simulink library "tp333079"  (Simulink 5.0)
values from neighbouring files (symbols this model uses):
  b = 1    [main_flock3.m]    (also in main_flock4.m; params_flocking_ros.m)
undefined symbols (not defined in the file or in its folder): AC, AlphaBnd, BetaBnd, CDda, CDde, CDdf, CDdr, CDM, CDmin, CGempty, CGgross, CL0, CLa, CLalphadot, Clbeta, Clda, CLde, CLdf, Cldr, CLM, CLmind, Clp, CLq, Clr, Cm0, Cma, Cmalphadot, Cmde, Cmdf, CmM, Cmq, Cnbeta, Cnda, Cndr, Cnp, Cnr, CP, CT, CYbeta, CYda, CYdr, CYp, CYr, Displacement, dmy, Engine, EulerIni, FuelFlow, FuelIni, J, Jempty, Jeng, Jgross, Jprop, MAC, MAP, MAPLim, MassIni, MaxPower, mempty ... (+26)
libraries: aerosimlib x325, simulink3 x42
(part 7 of 11)

== system tp333079/Equations of Motion/Geodetic-Frame EOM/Position ==
  note: Sources
  note: Position derivatives
  note: Navigation equation
  Vel NED : Inport  Port=1  PortDimensions=[3 1]  SampleTime=-1  DataType=auto
      settings: SignalType=auto
  Rmeridian : Inport  Port=2  PortDimensions=1  SampleTime=-1  DataType=auto
      settings: SignalType=auto
  Rnormal : Inport  Port=3  PortDimensions=1  SampleTime=-1  DataType=auto
      settings: SignalType=auto
  AConGnd : Inport  Port=4  PortDimensions=1  SampleTime=-1  DataType=auto
      settings: SignalType=auto
  RST : Inport  Port=5  PortDimensions=1  SampleTime=-1  DataType=auto
      settings: SignalType=auto
  Altitude Switch : Switch  Threshold=1
  ChSign : Gain  Gain=-1  Multiplication=Element-wise(K.*u)  SaturateOnIntegerOverflow=on
  Demux1 : Demux  Outputs=3  BusSelectionMode=off
  Demux3 : Demux  Outputs=3  BusSelectionMode=off
  Latitude Bound : Subsystem  SimViewingDevice=off
      settings: Permissions=ReadWrite  RTWFcnNameOpts=Auto  RTWFileNameOpts=Auto
      mask Type: Latitude bound
      mask Description: Bounds the latitude to [-pi/2, pi/2]. When the lower bound is exceeded the latitude is increasing again; when the upper bound is exceeded the latitude is decreasing.
  Longitude Bound : Subsystem  SimViewingDevice=off
      settings: Permissions=ReadWrite  RTWFcnNameOpts=Auto  RTWFileNameOpts=Auto
      mask Type: Longitude bound
      mask Description: Bounds the longitude to [-pi, pi]. When -pi bound is exceeded the longitude wraps back to pi; when the pi bound is exceeded the longitude wraps back to -pi.
  Mux : Mux  Inputs=3
  Mux1 : Mux  Inputs=3
  Position Integrator : Integrator  ExternalReset=rising  InitialConditionSource=internal  InitialCondition=PositionIni  LimitOutput=off  UpperSaturationLimit=inf  LowerSaturationLimit=-inf  ShowSaturationPort=off  ShowStatePort=off  AbsoluteTolerance=auto
  Sum : Sum  Inputs=|++  SaturateOnIntegerOverflow=on
  Sum1 : Sum  Inputs=|++  SaturateOnIntegerOverflow=on
  Ve/(Rn+h)cos(phi) : Product  Inputs=*//  Multiplication=Element-wise(.*)  SaturateOnIntegerOverflow=on
  Vn/(Rm+h) : Product  Inputs=*/  Multiplication=Element-wise(.*)  SaturateOnIntegerOverflow=on
  Zero : Constant  Value=0
  cos(phi) : Trigonometry  Operator=cos  OutputSignalType=auto
  Position : Outport  Port=1
  dPosdt : Outport  Port=2
  wires:
  Demux1/1 -> Vn/(Rm+h)/1
  Demux1/3 -> ChSign/1
  Demux1/2 -> Ve/(Rn+h)cos(phi)/1
  Vel NED/1 -> Demux1/1
  Rmeridian/1 -> Sum/1
  Rnormal/1 -> Sum1/1
  Sum/1 -> Vn/(Rm+h)/2
  Vn/(Rm+h)/1 -> Mux/1
  Sum1/1 -> Ve/(Rn+h)cos(phi)/2
  Ve/(Rn+h)cos(phi)/1 -> Mux/2
  AConGnd/1 -> Altitude Switch/2
  Zero/1 -> Altitude Switch/1
  ChSign/1 -> Altitude Switch/3
  Altitude Switch/1 -> Mux/3
  Mux/1 -> Position Integrator/1, dPosdt/1
  RST/1 -> Position Integrator/2
  Position Integrator/1 -> Demux3/1
  cos(phi)/1 -> Ve/(Rn+h)cos(phi)/3
  Demux3/3 -> Sum/2, Sum1/2, Mux1/3
  Demux3/2 -> Longitude Bound/1(In)
  Demux3/1 -> Latitude Bound/1(In)
  Longitude Bound/1(Out) -> Mux1/2
  Mux1/1 -> Position/1
  Latitude Bound/1(Out) -> cos(phi)/1, Mux1/1

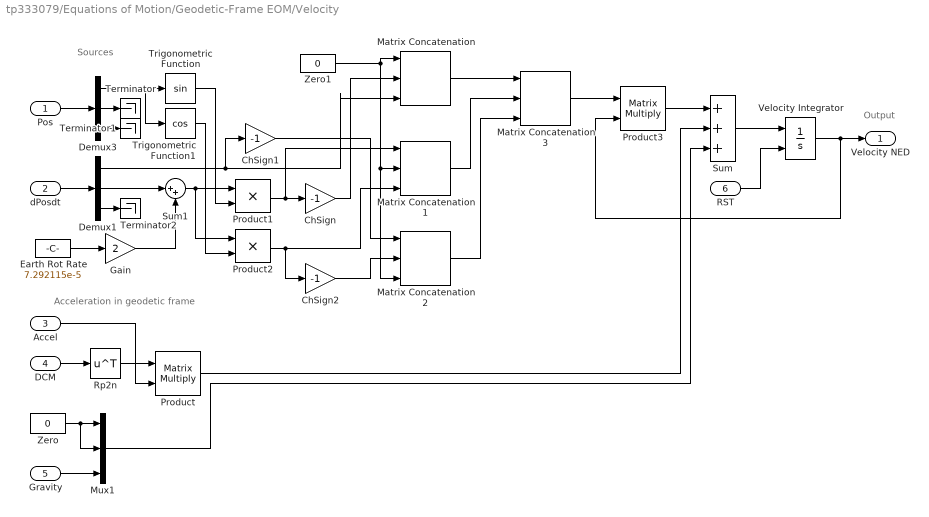
== system tp333079/Equations of Motion/Geodetic-Frame EOM/Velocity ==
  note: Sources
  note: Output
  note: Acceleration in geodetic frame
  Pos : Inport  Port=1  PortDimensions=[3 1]  SampleTime=-1  DataType=auto
      settings: SignalType=auto
  dPosdt : Inport  Port=2  PortDimensions=[3 1]  SampleTime=-1  DataType=auto
      settings: SignalType=auto
  Accel : Inport  Port=3  PortDimensions=[3 1]  SampleTime=-1  DataType=auto
      settings: SignalType=auto
  DCM : Inport  Port=4  PortDimensions=[3 3]  SampleTime=-1  DataType=auto
      settings: SignalType=auto
  Gravity : Inport  Port=5  PortDimensions=1  SampleTime=-1  DataType=auto
      settings: SignalType=auto
  RST : Inport  Port=6  PortDimensions=1  SampleTime=-1  DataType=auto
      settings: SignalType=auto
  ChSign : Gain  Gain=-1  Multiplication=Element-wise(K.*u)  SaturateOnIntegerOverflow=on
  ChSign1 : Gain  Gain=-1  Multiplication=Element-wise(K.*u)  SaturateOnIntegerOverflow=on
  ChSign2 : Gain  Gain=-1  Multiplication=Element-wise(K.*u)  SaturateOnIntegerOverflow=on
  Demux1 : Demux  Outputs=3  BusSelectionMode=off
  Demux3 : Demux  Outputs=3  BusSelectionMode=off
  Earth Rot Rate : Constant  Value=7.292115e-5
  Gain : Gain  Gain=2  Multiplication=Element-wise(K.*u)  SaturateOnIntegerOverflow=on
  Matrix Concatenation : simulink3/Signals & Systems/Matrix Concatenation  numInports=3  catMethod=Horizontal
  Matrix Concatenation1 : simulink3/Signals & Systems/Matrix Concatenation  numInports=3  catMethod=Horizontal
  Matrix Concatenation2 : simulink3/Signals & Systems/Matrix Concatenation  numInports=3  catMethod=Horizontal
  Matrix Concatenation3 : simulink3/Signals & Systems/Matrix Concatenation  numInports=3  catMethod=Vertical
  Mux1 : Mux  Inputs=3
  Product : Product  Inputs=2  Multiplication=Matrix(*)  SaturateOnIntegerOverflow=on
  Product1 : Product  Inputs=2  Multiplication=Element-wise(.*)  SaturateOnIntegerOverflow=on
  Product2 : Product  Inputs=2  Multiplication=Element-wise(.*)  SaturateOnIntegerOverflow=on
  Product3 : Product  Inputs=2  Multiplication=Matrix(*)  SaturateOnIntegerOverflow=on
  Rp2n : Math  Operator=transpose  OutputSignalType=auto
  Sum : Sum  Inputs=+++  SaturateOnIntegerOverflow=on
  Sum1 : Sum  Inputs=|++  SaturateOnIntegerOverflow=on
  Terminator : Terminator
  Terminator1 : Terminator
  Terminator2 : Terminator
  Trigonometric Function : Trigonometry  Operator=sin  OutputSignalType=auto
  Trigonometric Function1 : Trigonometry  Operator=cos  OutputSignalType=auto
  Velocity Integrator : Integrator  ExternalReset=rising  InitialConditionSource=internal  InitialCondition=VelocitiesIni  LimitOutput=off  UpperSaturationLimit=inf  LowerSaturationLimit=-inf  ShowSaturationPort=off  ShowStatePort=off  AbsoluteTolerance=auto
  Zero : Constant  Value=0
  Zero1 : Constant  Value=0
  Velocity NED : Outport  Port=1
  wires:
  Zero/1 -> Mux1/2, Mux1/1
  Gravity/1 -> Mux1/3
  Sum/1 -> Velocity Integrator/1
  RST/1 -> Velocity Integrator/2
  Velocity Integrator/1 -> Velocity NED/1, Product3/2
  DCM/1 -> Rp2n/1
  Rp2n/1 -> Product/1
  Accel/1 -> Product/2
  Pos/1 -> Demux3/1
  dPosdt/1 -> Demux1/1
  Earth Rot Rate/1 -> Gain/1
  Demux1/2 -> Sum1/1
  Gain/1 -> Sum1/2
  Demux3/1 -> Trigonometric Function/1, Trigonometric Function1/1
  Sum1/1 -> Product1/1, Product2/1
  Trigonometric Function/1 -> Product1/2
  Trigonometric Function1/1 -> Product2/2
  Zero1/1 -> Matrix Concatenation/1, Matrix Concatenation1/2, Matrix Concatenation2/3
  Product1/1 -> ChSign/1, Matrix Concatenation1/1
  ChSign/1 -> Matrix Concatenation/2
  Demux1/1 -> Matrix Concatenation/3, ChSign1/1
  Product2/1 -> Matrix Concatenation1/3, ChSign2/1
  ChSign1/1 -> Matrix Concatenation2/1
  ChSign2/1 -> Matrix Concatenation2/2
  Demux3/2 -> Terminator/1
  Demux3/3 -> Terminator1/1
  Demux1/3 -> Terminator2/1
  Matrix Concatenation/1 -> Matrix Concatenation3/1
  Matrix Concatenation1/1 -> Matrix Concatenation3/2
  Matrix Concatenation2/1 -> Matrix Concatenation3/3
  Matrix Concatenation3/1 -> Product3/1
  Product3/1 -> Sum/1
  Product/1 -> Sum/2
  Mux1/1 -> Sum/3

== system tp333079/Equations of Motion/Total Moment/Aero Moment ==
  Vec1 : Inport  Port=1  PortDimensions=-1  SampleTime=-1  DataType=auto
      settings: SignalType=auto
  Vec2 : Inport  Port=2  PortDimensions=-1  SampleTime=-1  DataType=auto
      settings: SignalType=auto
  Product : Product  Inputs=2  Multiplication=Element-wise(.*)  SaturateOnIntegerOverflow=on
  Product1 : Product  Inputs=2  Multiplication=Element-wise(.*)  SaturateOnIntegerOverflow=on
  Selector : Selector  InputType=Vector  ElementSrc=Internal  Elements=[2 3 1]  RowSrc=Internal  Rows=1  ColumnSrc=Internal  Columns=1  InputPortWidth=3
  Selector1 : Selector  InputType=Vector  ElementSrc=Internal  Elements=[3 1 2]  RowSrc=Internal  Rows=1  ColumnSrc=Internal  Columns=1  InputPortWidth=3
  Selector2 : Selector  InputType=Vector  ElementSrc=Internal  Elements=[3 1 2]  RowSrc=Internal  Rows=1  ColumnSrc=Internal  Columns=1  InputPortWidth=3
  Selector3 : Selector  InputType=Vector  ElementSrc=Internal  Elements=[2 3 1]  RowSrc=Internal  Rows=1  ColumnSrc=Internal  Columns=1  InputPortWidth=3
  Sum : Sum  Inputs=+-  SaturateOnIntegerOverflow=on
  ProdVec : Outport  Port=1
  wires:
  Sum/1 -> ProdVec/1
  Product1/1 -> Sum/2
  Product/1 -> Sum/1
  Selector3/1 -> Product1/2
  Selector2/1 -> Product1/1
  Selector1/1 -> Product/2
  Selector/1 -> Product/1
  Vec2/1 -> Selector3/1, Selector1/1
  Vec1/1 -> Selector2/1, Selector/1

== system tp333079/Equations of Motion/Total Moment/Propulsion Moment ==
  Vec1 : Inport  Port=1  PortDimensions=-1  SampleTime=-1  DataType=auto
      settings: SignalType=auto
  Vec2 : Inport  Port=2  PortDimensions=-1  SampleTime=-1  DataType=auto
      settings: SignalType=auto
  Product : Product  Inputs=2  Multiplication=Element-wise(.*)  SaturateOnIntegerOverflow=on
  Product1 : Product  Inputs=2  Multiplication=Element-wise(.*)  SaturateOnIntegerOverflow=on
  Selector : Selector  InputType=Vector  ElementSrc=Internal  Elements=[2 3 1]  RowSrc=Internal  Rows=1  ColumnSrc=Internal  Columns=1  InputPortWidth=3
  Selector1 : Selector  InputType=Vector  ElementSrc=Internal  Elements=[3 1 2]  RowSrc=Internal  Rows=1  ColumnSrc=Internal  Columns=1  InputPortWidth=3
  Selector2 : Selector  InputType=Vector  ElementSrc=Internal  Elements=[3 1 2]  RowSrc=Internal  Rows=1  ColumnSrc=Internal  Columns=1  InputPortWidth=3
  Selector3 : Selector  InputType=Vector  ElementSrc=Internal  Elements=[2 3 1]  RowSrc=Internal  Rows=1  ColumnSrc=Internal  Columns=1  InputPortWidth=3
  Sum : Sum  Inputs=+-  SaturateOnIntegerOverflow=on
  ProdVec : Outport  Port=1
  wires:
  Vec1/1 -> Selector/1, Selector2/1
  Vec2/1 -> Selector1/1, Selector3/1
  Selector/1 -> Product/1
  Selector1/1 -> Product/2
  Selector2/1 -> Product1/1
  Selector3/1 -> Product1/2
  Product/1 -> Sum/1
  Product1/1 -> Sum/2
  Sum/1 -> ProdVec/1

== system tp333079/FlightGear-Compatible/Aerodynamics/Coefficient ==
  RowParam : Inport  Port=1  PortDimensions=-1  SampleTime=-1  DataType=auto
      settings: SignalType=auto
  ColParam : Inport  Port=2  PortDimensions=-1  SampleTime=-1  DataType=auto
      settings: SignalType=auto
  Value : aerosimlib/FlightGear-Compatible/Aerodynamics/Value  Value=0
  term2 : Terminator
  Coeff : Outport  Port=1
  wires:
  RowParam/1 -> Value/1
  Value/1 -> Coeff/1
  ColParam/1 -> term2/1

== system tp333079/FlightGear-Compatible/Aerodynamics/Table ==
  RowParam : Inport  Port=1  PortDimensions=-1  SampleTime=-1  DataType=auto
      settings: SignalType=auto
  ColParam : Inport  Port=2  PortDimensions=-1  SampleTime=-1  DataType=auto
      settings: SignalType=auto
  Look-Up Table (2-D) : Lookup2D  RowIndex=Table.RowArg  ColumnIndex=Table.ColArg  OutputValues=Table.Data
  Coeff : Outport  Port=1
  wires:
  Look-Up Table (2-D)/1 -> Coeff/1
  ColParam/1 -> Look-Up Table (2-D)/2
  RowParam/1 -> Look-Up Table (2-D)/1

== system tp333079/FlightGear-Compatible/Aerodynamics/Value ==
  RowParam : Inport  Port=1  PortDimensions=-1  SampleTime=-1  DataType=auto
      settings: SignalType=auto
  Gain : Gain  Gain=Value.Data  Multiplication=Element-wise(K.*u)  SaturateOnIntegerOverflow=on
  Coeff : Outport  Port=1
  wires:
  RowParam/1 -> Gain/1
  Gain/1 -> Coeff/1

== system tp333079/FlightGear-Compatible/Aerodynamics/Vector ==
  RowParam : Inport  Port=1  PortDimensions=-1  SampleTime=-1  DataType=auto
      settings: SignalType=auto
  Look-Up Table : Lookup  InputValues=Vector.RowArg  OutputValues=Vector.Data
  Coeff : Outport  Port=1
  wires:
  RowParam/1 -> Look-Up Table/1
  Look-Up Table/1 -> Coeff/1

== system tp333079/FlightGear-Compatible/Complete Aircraft/CESSNA-172 ==
  Control : Inport  Port=1  PortDimensions=[7 1]  SampleTime=-1  DataType=auto
      settings: SignalType=auto
  Wind : Inport  Port=2  PortDimensions=[3 1]  SampleTime=-1  DataType=auto
      settings: SignalType=auto
  RST : Inport  Port=3  PortDimensions=1  SampleTime=-1  DataType=auto
      settings: SignalType=auto
  Aerodynamics : Subsystem  SimViewingDevice=off
      settings: Permissions=ReadWrite  RTWFcnNameOpts=Auto  RTWFileNameOpts=Auto
  Aircraft Inertia : Subsystem  SimViewingDevice=off
      settings: Permissions=ReadWrite  RTWFcnNameOpts=Auto  RTWFileNameOpts=Auto
  Atmosphere : Subsystem  SimViewingDevice=off
      settings: Permissions=ReadWrite  RTWFcnNameOpts=Auto  RTWFileNameOpts=Auto
  Demux : Demux  Outputs=7  BusSelectionMode=off
  Demux1 : Demux  Outputs=3  BusSelectionMode=off
  Earth : Subsystem  SimViewingDevice=off
      settings: Permissions=ReadWrite  RTWFcnNameOpts=Auto  RTWFileNameOpts=Auto
  Equations of Motion : Subsystem  SimViewingDevice=off
      settings: Permissions=ReadWrite  RTWFcnNameOpts=Auto  RTWFileNameOpts=Auto
  F/m : Product  Inputs=*/  Multiplication=Element-wise(.*)  SaturateOnIntegerOverflow=on
  Mux : Mux  Inputs=4
  Mux1 : Mux  Inputs=3
  Propulsion System : aerosimlib/FlightGear-Compatible/Propulsion/FG Piston Engine +  Fixed-Pitch Prop  Eng=AC.Propulsion.Engine{1}  Thr=AC.Propulsion.Thruster{1}  pSL=101325  TSL=288.15  OmegaIni=OmegaIni
  Sum1 : Sum  Inputs=++  SaturateOnIntegerOverflow=on
  Sum2 : Sum  Inputs=++  SaturateOnIntegerOverflow=on
  rad/s 2 RPM : aerosimlib/Unit Conversion/Angular velocity/rad//s 2 RPM
  TAS : Outport  Port=1
  AOA : Outport  Port=2
  Position : Outport  Port=3
  Attitude : Outport  Port=4
  Rates : Outport  Port=5
  Aero : Outport  Port=6
  Prop : Outport  Port=7
  Engine : Outport  Port=8
  RPM : Outport  Port=9
  wires:
  rad/s 2 RPM/1 -> RPM/1
  Propulsion System/3 -> rad/s 2 RPM/1
  Propulsion System/5 -> Engine/1
  Propulsion System/6 -> Prop/1
  Aerodynamics/3(AeroCoeff) -> Aero/1
  Equations of Motion/7(Euler) -> Attitude/1
  Demux1/3 -> AOA/1
  Demux1/1 -> TAS/1
  Equations of Motion/6(DCM) -> Atmosphere/6(DCM)
  Equations of Motion/1(VelB) -> Atmosphere/4(VelB), Aerodynamics/2(VelB)
  Equations of Motion/3(Rates) -> Rates/1, Aerodynamics/4(Rates)
  Earth/2(AGL) -> Aerodynamics/8(AGL), Atmosphere/2(AGL)
  Earth/1(MSL) -> Atmosphere/1(MSL)
  Earth/3(AConGnd) -> Equations of Motion/6(AConGnd)
  Earth/6(Gravity) -> Equations of Motion/5(Gravity)
  Earth/4(Rearth) -> Equations of Motion/4(Rearth)
  Equations of Motion/5(Pos) -> Position/1, Earth/1(Position)
  Aircraft Inertia/3(Inertia) -> Equations of Motion/3(Inertia)
  Aircraft Inertia/2(CG) -> Propulsion System/6, Aerodynamics/9(CGpos)
  Aircraft Inertia/1(Mass) -> F/m/2
  Propulsion System/4 -> Aircraft Inertia/1(FuelFlow)
  RST/1 -> Aircraft Inertia/2(RST), Equations of Motion/7(RST), Propulsion System/7
  Aerodynamics/4(VelW) -> Demux1/1, Atmosphere/5(VelW), Propulsion System/5
  Atmosphere/2(OAT) -> Propulsion System/3
  Atmosphere/1(pstatic) -> Propulsion System/2
  Atmosphere/5(WindVel) -> Aerodynamics/3(WindB)
  Atmosphere/6(WindRates) -> Aerodynamics/5(WindRates)
  Wind/1 -> Atmosphere/3(Winds)
  Atmosphere/4(a) -> Aerodynamics/7(a)
  Atmosphere/3(rho) -> Propulsion System/4, Aerodynamics/6(rho)
  Mux1/1 -> Propulsion System/1
  Mux/1 -> Aerodynamics/1(Control)
  Control/1 -> Demux/1
  Demux/7 -> Mux1/3
  Demux/6 -> Mux1/2
  Demux/5 -> Mux1/1
  Demux/4 -> Mux/4
  Demux/3 -> Mux/3
  Demux/2 -> Mux/2
  Demux/1 -> Mux/1
  F/m/1 -> Equations of Motion/1(Accel)
  Sum2/1 -> F/m/1
  Sum1/1 -> Equations of Motion/2(Moment)
  Aerodynamics/1(Faero) -> Sum2/1
  Propulsion System/1 -> Sum2/2
  Propulsion System/2 -> Sum1/2
  Aerodynamics/2(Maero) -> Sum1/1

== system tp333079/FlightGear-Compatible/Complete Aircraft/CESSNA-182 ==
  Control : Inport  Port=1  PortDimensions=[8 1]  SampleTime=-1  DataType=auto
      settings: SignalType=auto
  Wind : Inport  Port=2  PortDimensions=[3 1]  SampleTime=-1  DataType=auto
      settings: SignalType=auto
  RST : Inport  Port=3  PortDimensions=1  SampleTime=-1  DataType=auto
      settings: SignalType=auto
  Aerodynamics : Subsystem  SimViewingDevice=off
      settings: Permissions=ReadWrite  RTWFcnNameOpts=Auto  RTWFileNameOpts=Auto
  Aircraft Inertia : Subsystem  SimViewingDevice=off
      settings: Permissions=ReadWrite  RTWFcnNameOpts=Auto  RTWFileNameOpts=Auto
  Atmosphere : aerosimlib/FlightGear-Compatible/Complete Aircraft/CESSNA-172/Atmosphere  SimViewingDevice=off
      settings: Permissions=ReadWrite  RTWFcnNameOpts=Auto  RTWFileNameOpts=Auto
  Demux : Demux  Outputs=8  BusSelectionMode=off
  Demux1 : Demux  Outputs=3  BusSelectionMode=off
  Earth : Subsystem  SimViewingDevice=off
      settings: Permissions=ReadWrite  RTWFcnNameOpts=Auto  RTWFileNameOpts=Auto
  Equations of Motion : Subsystem  SimViewingDevice=off
      settings: Permissions=ReadWrite  RTWFcnNameOpts=Auto  RTWFileNameOpts=Auto
  F/m : Product  Inputs=*/  Multiplication=Element-wise(.*)  SaturateOnIntegerOverflow=on
  FG Piston Engine +  Variable-Pitch Prop : aerosimlib/FlightGear-Compatible/Propulsion/FG Piston Engine +  Variable-Pitch Prop  Eng=AC.Propulsion.Engine{1}  Thr=AC.Propulsion.Thruster{1}  pSL=101325  TSL=288.15  OmegaIni=OmegaIni
  Mux : Mux  Inputs=4
  Mux1 : Mux  Inputs=4
  Sum1 : Sum  Inputs=++  SaturateOnIntegerOverflow=on
  Sum2 : Sum  Inputs=++  SaturateOnIntegerOverflow=on
  rad/s 2 RPM : aerosimlib/Unit Conversion/Angular velocity/rad//s 2 RPM
  TAS : Outport  Port=1
  AOA : Outport  Port=2
  Position : Outport  Port=3
  Attitude : Outport  Port=4
  Rates : Outport  Port=5
  Aero : Outport  Port=6
  Prop : Outport  Port=7
  Engine : Outport  Port=8
  RPM : Outport  Port=9
  wires:
  Demux/8 -> Mux1/4
  rad/s 2 RPM/1 -> RPM/1
  FG Piston Engine +  Variable-Pitch Prop/3 -> rad/s 2 RPM/1
  FG Piston Engine +  Variable-Pitch Prop/5 -> Engine/1
  FG Piston Engine +  Variable-Pitch Prop/6 -> Prop/1
  Aerodynamics/3(AeroCoeff) -> Aero/1
  Equations of Motion/7(Euler) -> Attitude/1
  Demux1/3 -> AOA/1
  Demux1/1 -> TAS/1
  Equations of Motion/6(DCM) -> Atmosphere/6
  Equations of Motion/1(VelB) -> Aerodynamics/2(VelB), Atmosphere/4
  Equations of Motion/3(Rates) -> Rates/1, Aerodynamics/4(Rates)
  Earth/2(AGL) -> Aerodynamics/8(AGL), Atmosphere/2
  Earth/1(MSL) -> Atmosphere/1
  Earth/3(AConGnd) -> Equations of Motion/6(AConGnd)
  Earth/6(Gravity) -> Equations of Motion/5(Gravity)
  Earth/4(Rearth) -> Equations of Motion/4(Rearth)
  Equations of Motion/5(Pos) -> Position/1, Earth/1(Position)
  Aircraft Inertia/3(Inertia) -> Equations of Motion/3(Inertia)
  F/m/1 -> Equations of Motion/1(Accel)
  Aircraft Inertia/2(CG) -> FG Piston Engine +  Variable-Pitch Prop/6, Aerodynamics/9(CGpos)
  Aircraft Inertia/1(Mass) -> F/m/2
  FG Piston Engine +  Variable-Pitch Prop/4 -> Aircraft Inertia/1(FuelFlow)
  RST/1 -> Aircraft Inertia/2(RST), Equations of Motion/7(RST), FG Piston Engine +  Variable-Pitch Prop/7
  Aerodynamics/4(VelW) -> Demux1/1, FG Piston Engine +  Variable-Pitch Prop/5, Atmosphere/5
  Atmosphere/2 -> FG Piston Engine +  Variable-Pitch Prop/3
  Atmosphere/1 -> FG Piston Engine +  Variable-Pitch Prop/2
  Atmosphere/5 -> Aerodynamics/3(WindB)
  Atmosphere/6 -> Aerodynamics/5(WindRates)
  Wind/1 -> Atmosphere/3
  Atmosphere/4 -> Aerodynamics/7(a)
  Atmosphere/3 -> FG Piston Engine +  Variable-Pitch Prop/4, Aerodynamics/6(rho)
  Mux1/1 -> FG Piston Engine +  Variable-Pitch Prop/1
  Mux/1 -> Aerodynamics/1(Control)
  Control/1 -> Demux/1
  Demux/7 -> Mux1/3
  Demux/6 -> Mux1/2
  Demux/5 -> Mux1/1
  Demux/4 -> Mux/4
  Demux/3 -> Mux/3
  Demux/2 -> Mux/2
  Demux/1 -> Mux/1
  FG Piston Engine +  Variable-Pitch Prop/2 -> Sum1/2
  Sum2/1 -> F/m/1
  Sum1/1 -> Equations of Motion/2(Moment)
  Aerodynamics/1(Faero) -> Sum2/1
  Aerodynamics/2(Maero) -> Sum1/1
  FG Piston Engine +  Variable-Pitch Prop/1 -> Sum2/2

== system tp333079/FlightGear-Compatible/Complete Aircraft/CESSNA-310 ==
  Control : Inport  Port=1  PortDimensions=[12 1]  SampleTime=-1  DataType=auto
      settings: SignalType=auto
  Gear : Inport  Port=2  PortDimensions=1  SampleTime=-1  DataType=auto
      settings: SignalType=auto
  Wind : Inport  Port=3  PortDimensions=[3 1]  SampleTime=-1  DataType=auto
      settings: SignalType=auto
  RST : Inport  Port=4  PortDimensions=1  SampleTime=-1  DataType=auto
      settings: SignalType=auto
  Aerodynamics : Subsystem  SimViewingDevice=off
      settings: Permissions=ReadWrite  RTWFcnNameOpts=Auto  RTWFileNameOpts=Auto
  Aircraft Inertia : Subsystem  SimViewingDevice=off
      settings: Permissions=ReadWrite  RTWFcnNameOpts=Auto  RTWFileNameOpts=Auto
  Atmosphere : aerosimlib/FlightGear-Compatible/Complete Aircraft/CESSNA-172/Atmosphere  SimViewingDevice=off
      settings: Permissions=ReadWrite  RTWFcnNameOpts=Auto  RTWFileNameOpts=Auto
  Demux : Demux  Outputs=3  BusSelectionMode=off
  Demux1 : Demux  Outputs=3  BusSelectionMode=off
  Earth : Subsystem  SimViewingDevice=off
      settings: Permissions=ReadWrite  RTWFcnNameOpts=Auto  RTWFileNameOpts=Auto
  Equations of Motion : Subsystem  SimViewingDevice=off
      settings: Permissions=ReadWrite  RTWFcnNameOpts=Auto  RTWFileNameOpts=Auto
  F/m : Product  Inputs=*/  Multiplication=Element-wise(.*)  SaturateOnIntegerOverflow=on
  Left Engine : aerosimlib/FlightGear-Compatible/Propulsion/FG Piston Engine +  Variable-Pitch Prop  Eng=AC.Propulsion.Engine{1}  Thr=AC.Propulsion.Thruster{1}  pSL=101325  TSL=288.15  OmegaIni=OmegaIni(1)
  Right Engine : aerosimlib/FlightGear-Compatible/Propulsion/FG Piston Engine +  Variable-Pitch Prop  Eng=AC.Propulsion.Engine{2}  Thr=AC.Propulsion.Thruster{2}  pSL=101325  TSL=288.15  OmegaIni=OmegaIni(2)
  Sum : Sum  Orientation=left  Inputs=|++  SaturateOnIntegerOverflow=on
  Sum1 : Sum  Inputs=+++  SaturateOnIntegerOverflow=on
  Sum2 : Sum  Inputs=+++  SaturateOnIntegerOverflow=on
  rad/s 2 RPM : aerosimlib/Unit Conversion/Angular velocity/rad//s 2 RPM
  rad/s 2 RPM1 : aerosimlib/Unit Conversion/Angular velocity/rad//s 2 RPM
  TAS : Outport  Port=1
  AOA : Outport  Port=2
  Position : Outport  Port=3
  Attitude : Outport  Port=4
  Rates : Outport  Port=5
  Aero : Outport  Port=6
  PropL : Outport  Port=7
  EngineL : Outport  Port=8
  RPML : Outport  Port=9
  PropR : Outport  Port=10
  EngineR : Outport  Port=11
  RPMR : Outport  Port=12
  wires:
  Gear/1 -> Aerodynamics/10(Gear)
  Demux/1 -> Aerodynamics/1(Control)
  Earth/1(MSL) -> Atmosphere/1
  Equations of Motion/6(DCM) -> Atmosphere/6
  Earth/2(AGL) -> Aerodynamics/8(AGL), Atmosphere/2
  Atmosphere/4 -> Aerodynamics/7(a)
  Atmosphere/6 -> Aerodynamics/5(WindRates)
  Atmosphere/5 -> Aerodynamics/3(WindB)
  Equations of Motion/1(VelB) -> Aerodynamics/2(VelB), Atmosphere/4
  rad/s 2 RPM1/1 -> RPMR/1
  Right Engine/5 -> EngineR/1
  Right Engine/6 -> PropR/1
  rad/s 2 RPM/1 -> RPML/1
  Left Engine/6 -> PropL/1
  Left Engine/5 -> EngineL/1
  Right Engine/3 -> rad/s 2 RPM1/1
  Left Engine/3 -> rad/s 2 RPM/1
  Right Engine/2 -> Sum2/2
  Left Engine/2 -> Sum2/3
  Aerodynamics/2(Maero) -> Sum2/1
  Sum2/1 -> Equations of Motion/2(Moment)
  Right Engine/1 -> Sum1/2
  Left Engine/1 -> Sum1/3
  Aircraft Inertia/1(Mass) -> F/m/2
  Sum1/1 -> F/m/1
  F/m/1 -> Equations of Motion/1(Accel)
  Sum/1 -> Aircraft Inertia/1(FuelFlow)
  Left Engine/4 -> Sum/2
  Right Engine/4 -> Sum/1
  Atmosphere/3 -> Aerodynamics/6(rho), Right Engine/4, Left Engine/4
  Atmosphere/2 -> Right Engine/3, Left Engine/3
  Atmosphere/1 -> Right Engine/2, Left Engine/2
  Demux/3 -> Right Engine/1
  Demux/2 -> Left Engine/1
  Wind/1 -> Atmosphere/3
  Aerodynamics/3(AeroCoeff) -> Aero/1
  Equations of Motion/7(Euler) -> Attitude/1
  Demux1/3 -> AOA/1
  Demux1/1 -> TAS/1
  Equations of Motion/3(Rates) -> Rates/1, Aerodynamics/4(Rates)
  Earth/3(AConGnd) -> Equations of Motion/6(AConGnd)
  Earth/6(Gravity) -> Equations of Motion/5(Gravity)
  Earth/4(Rearth) -> Equations of Motion/4(Rearth)
  Equations of Motion/5(Pos) -> Position/1, Earth/1(Position)
  Aircraft Inertia/3(Inertia) -> Equations of Motion/3(Inertia)
  Aircraft Inertia/2(CG) -> Left Engine/6, Aerodynamics/9(CGpos), Right Engine/6
  Aerodynamics/1(Faero) -> Sum1/1
  RST/1 -> Right Engine/7, Left Engine/7, Aircraft Inertia/2(RST), Equations of Motion/7(RST)
  Aerodynamics/4(VelW) -> Right Engine/5, Left Engine/5, Atmosphere/5, Demux1/1
  Control/1 -> Demux/1

== system tp333079/FlightGear-Compatible/Inertia/Empty Aircraft ==
  ACMass : Constant  Value=Metrics.EmptyWeight
  CG Location : Constant  Value=Metrics.CGLoc
  Moments of Inertia : Constant  Value=[Metrics.InertiaX Metrics.InertiaY Metrics.InertiaZ Metrics.InertiaXZ]
  Mass : Outport  Port=1
  CG : Outport  Port=2
  Inertia : Outport  Port=3
  wires:
  ACMass/1 -> Mass/1
  CG Location/1 -> CG/1
  Moments of Inertia/1 -> Inertia/1

== system tp333079/FlightGear-Compatible/Inertia/Point Mass ==
  J1 : Product  Inputs=2  Multiplication=Element-wise(.*)  SaturateOnIntegerOverflow=on
  J2 : Product  Inputs=2  Multiplication=Element-wise(.*)  SaturateOnIntegerOverflow=on
  J3 : Product  Inputs=2  Multiplication=Element-wise(.*)  SaturateOnIntegerOverflow=on
  Jxz : Product  Inputs=3  Multiplication=Element-wise(.*)  SaturateOnIntegerOverflow=on
  M : Constant  Value=PointMass(1)
  Math Function1 : Math  Operator=square  OutputSignalType=auto
  Math Function2 : Math  Operator=square  OutputSignalType=auto
  Math Function3 : Math  Operator=square  OutputSignalType=auto
  Mux : Mux  Inputs=3
  Mux1 : Mux  Inputs=4
  Sum : Sum  Inputs=++  SaturateOnIntegerOverflow=on
  Sum1 : Sum  Inputs=++  SaturateOnIntegerOverflow=on
  Sum2 : Sum  Inputs=++  SaturateOnIntegerOverflow=on
  x pos : Constant  Value=PointMass(2)
  y pos : Constant  Value=PointMass(3)
  z pos : Constant  Value=PointMass(4)
  Mass : Outport  Port=1
  CG : Outport  Port=2
  Inertia : Outport  Port=3
  wires:
  J3/1 -> Mux1/3
  J2/1 -> Mux1/2
  J1/1 -> Mux1/1
  Mux1/1 -> Inertia/1
  Jxz/1 -> Mux1/4
  Mux/1 -> CG/1
  Sum/1 -> J3/2
  Sum2/1 -> J2/2
  Sum1/1 -> J1/2
  Math Function3/1 -> Sum2/2, Sum1/2
  Math Function2/1 -> Sum1/1, Sum/2
  Math Function1/1 -> Sum2/1, Sum/1
  z pos/1 -> Math Function3/1, Mux/3, Jxz/3
  y pos/1 -> Mux/2, Math Function2/1
  x pos/1 -> Mux/1, Jxz/2, Math Function1/1
  M/1 -> Mass/1, J1/1, J2/1, J3/1, Jxz/1

== system tp333079/FlightGear-Compatible/Propulsion/Engine ==
  Piston : Subsystem  SimViewingDevice=off
      settings: Permissions=ReadWrite  RTWFcnNameOpts=Auto  RTWFileNameOpts=Auto

== system tp333079/FlightGear-Compatible/Propulsion/FG Piston Engine +  Fixed-Pitch Prop ==
  Control : Inport  Port=1  PortDimensions=[3 1]  SampleTime=-1  DataType=double
      settings: SignalType=auto
  p : Inport  Port=2  PortDimensions=1  SampleTime=-1  DataType=double
      settings: SignalType=auto
  T : Inport  Port=3  PortDimensions=1  SampleTime=-1  DataType=double
      settings: SignalType=auto
  rho : Inport  Port=4  PortDimensions=1  SampleTime=-1  DataType=double
      settings: SignalType=auto
  WindAxesVel : Inport  Port=5  PortDimensions=[3 1]  SampleTime=-1  DataType=auto
      settings: SignalType=auto
  CGpos : Inport  Port=6  PortDimensions=[3 1]  SampleTime=-1  DataType=auto
      settings: SignalType=auto
  RST : Inport  Port=7  PortDimensions=1  SampleTime=-1  DataType=double
      settings: SignalType=auto
  ChSign : Gain  Gain=-Thr.Sense  Multiplication=Element-wise(K.*u)  SaturateOnIntegerOverflow=on
  Demux : Demux  Outputs=3  BusSelectionMode=off
  Demux1 : Demux  Outputs=3  BusSelectionMode=off
  Engine speed Integrator : Integrator  ExternalReset=rising  InitialConditionSource=internal  InitialCondition=OmegaIni  LimitOutput=on  UpperSaturationLimit=inf  LowerSaturationLimit=0  ShowSaturationPort=off  ShowStatePort=off  AbsoluteTolerance=auto
  FG Fixed-Pitch Propeller : aerosimlib/FlightGear-Compatible/Propulsion/Thruster/Propeller/FG Fixed-Pitch Propeller  Thr=Thr
  FG Piston Engine : aerosimlib/FlightGear-Compatible/Propulsion/Engine/Piston/FG Piston Engine  Eng=Eng  pSL=pSL  TSL=TSL
  M/J : Product  Inputs=*/  Multiplication=Element-wise(.*)  SaturateOnIntegerOverflow=on
  Mux : Mux  Inputs=3
  Mux1 : Mux  Inputs=3
  Mux2 : Mux  Inputs=5
  Propeller  moment of inertia : Constant  Value=Thr.Param.Inertia
  Sum : Sum  Inputs=|+-  SaturateOnIntegerOverflow=on
  Sum1 : Sum  Inputs=++  SaturateOnIntegerOverflow=on
  Sum2 : Sum  Inputs=|++  SaturateOnIntegerOverflow=on
  Terminator : Terminator
  Terminator1 : Terminator
  Zero : Constant  Value=0
  r x F : aerosimlib/Math/Cross Product
  r_prop : Constant  Value=Thr.Loc
  Fprop : Outport  Port=1
  Mprop : Outport  Port=2
  Omega : Outport  Port=3
  FuelFlow : Outport  Port=4
  EngCoeff : Outport  Port=5
  PropCoeff : Outport  Port=6
  wires:
  Control/1 -> Demux/1
  WindAxesVel/1 -> Demux1/1
  Demux1/2 -> Terminator/1
  Demux1/3 -> Terminator1/1
  Demux1/1 -> FG Fixed-Pitch Propeller/1
  rho/1 -> FG Piston Engine/6, FG Fixed-Pitch Propeller/2
  Propeller  moment of inertia/1 -> M/J/2
  FG Fixed-Pitch Propeller/2 -> Sum1/2
  Sum1/1 -> M/J/1
  M/J/1 -> Engine speed Integrator/1
  RST/1 -> Engine speed Integrator/2
  Engine speed Integrator/1 -> FG Piston Engine/3, FG Fixed-Pitch Propeller/3, Omega/1
  Zero/1 -> Mux/2, Mux/3, Mux1/3, Mux1/2
  FG Fixed-Pitch Propeller/1 -> Mux/1
  ChSign/1 -> Mux1/1
  FG Fixed-Pitch Propeller/3 -> PropCoeff/1
  Demux/1 -> FG Piston Engine/1
  Demux/2 -> FG Piston Engine/2
  p/1 -> FG Piston Engine/4
  T/1 -> FG Piston Engine/5
  FG Piston Engine/6 -> ChSign/1, Sum1/1
  FG Piston Engine/1 -> Mux2/1
  FG Piston Engine/2 -> Mux2/2
  FG Piston Engine/3 -> Mux2/3, FuelFlow/1
  FG Piston Engine/4 -> Mux2/4
  FG Piston Engine/5 -> Mux2/5
  Mux2/1 -> EngCoeff/1
  r_prop/1 -> Sum/1
  CGpos/1 -> Sum/2
  Sum/1 -> r x F/1
  Mux/1 -> r x F/2, Fprop/1
  Mux1/1 -> Sum2/1
  r x F/1 -> Sum2/2
  Sum2/1 -> Mprop/1

== system tp333079/FlightGear-Compatible/Propulsion/FG Piston Engine +  Variable-Pitch Prop ==
  Control : Inport  Port=1  PortDimensions=[4 1]  SampleTime=-1  DataType=double
      settings: SignalType=auto
  p : Inport  Port=2  PortDimensions=1  SampleTime=-1  DataType=double
      settings: SignalType=auto
  T : Inport  Port=3  PortDimensions=1  SampleTime=-1  DataType=double
      settings: SignalType=auto
  rho : Inport  Port=4  PortDimensions=1  SampleTime=-1  DataType=double
      settings: SignalType=auto
  WindAxesVel : Inport  Port=5  PortDimensions=[3 1]  SampleTime=-1  DataType=auto
      settings: SignalType=auto
  CGpos : Inport  Port=6  PortDimensions=[3 1]  SampleTime=-1  DataType=auto
      settings: SignalType=auto
  RST : Inport  Port=7  PortDimensions=1  SampleTime=-1  DataType=double
      settings: SignalType=auto
  ChSign : Gain  Gain=-Thr.Sense  Multiplication=Element-wise(K.*u)  SaturateOnIntegerOverflow=on
  Demux : Demux  Outputs=4  BusSelectionMode=off
  Demux1 : Demux  Outputs=3  BusSelectionMode=off
  Engine speed Integrator : Integrator  ExternalReset=rising  InitialConditionSource=internal  InitialCondition=OmegaIni  LimitOutput=on  UpperSaturationLimit=inf  LowerSaturationLimit=0  ShowSaturationPort=off  ShowStatePort=off  AbsoluteTolerance=auto
  FG Piston Engine : aerosimlib/FlightGear-Compatible/Propulsion/Engine/Piston/FG Piston Engine  Eng=Eng  pSL=pSL  TSL=TSL
  FG Variable-Pitch Propeller : aerosimlib/FlightGear-Compatible/Propulsion/Thruster/Propeller/FG Variable-Pitch Propeller  Thr=Thr
  M/J : Product  Inputs=*/  Multiplication=Element-wise(.*)  SaturateOnIntegerOverflow=on
  Mux : Mux  Inputs=3
  Mux1 : Mux  Inputs=3
  Mux2 : Mux  Inputs=5
  Propeller  moment of inertia : Constant  Value=Thr.Param.Inertia
  Sum : Sum  Inputs=|+-  SaturateOnIntegerOverflow=on
  Sum1 : Sum  Inputs=++  SaturateOnIntegerOverflow=on
  Sum2 : Sum  Inputs=|++  SaturateOnIntegerOverflow=on
  Terminator : Terminator
  Terminator1 : Terminator
  Zero : Constant  Value=0
  r x F : aerosimlib/Math/Cross Product
  r_prop : Constant  Value=Thr.Loc
  Fprop : Outport  Port=1
  Mprop : Outport  Port=2
  Omega : Outport  Port=3
  FuelFlow : Outport  Port=4
  EngCoeff : Outport  Port=5
  PropCoeff : Outport  Port=6
  wires:
  Demux/4 -> FG Variable-Pitch Propeller/4
  Control/1 -> Demux/1
  WindAxesVel/1 -> Demux1/1
  Demux1/2 -> Terminator/1
  Demux1/3 -> Terminator1/1
  Demux1/1 -> FG Variable-Pitch Propeller/1
  rho/1 -> FG Variable-Pitch Propeller/2, FG Piston Engine/6
  Propeller  moment of inertia/1 -> M/J/2
  FG Variable-Pitch Propeller/2 -> Sum1/2
  Sum1/1 -> M/J/1
  M/J/1 -> Engine speed Integrator/1
  RST/1 -> Engine speed Integrator/2
  Engine speed Integrator/1 -> FG Variable-Pitch Propeller/3, FG Piston Engine/3, Omega/1
  Zero/1 -> Mux/2, Mux/3, Mux1/3, Mux1/2
  FG Variable-Pitch Propeller/1 -> Mux/1
  ChSign/1 -> Mux1/1
  FG Variable-Pitch Propeller/3 -> PropCoeff/1
  Demux/1 -> FG Piston Engine/1
  Demux/2 -> FG Piston Engine/2
  p/1 -> FG Piston Engine/4
  T/1 -> FG Piston Engine/5
  FG Piston Engine/6 -> ChSign/1, Sum1/1
  FG Piston Engine/1 -> Mux2/1
  FG Piston Engine/2 -> Mux2/2
  FG Piston Engine/3 -> Mux2/3, FuelFlow/1
  FG Piston Engine/4 -> Mux2/4
  FG Piston Engine/5 -> Mux2/5
  Mux2/1 -> EngCoeff/1
  r_prop/1 -> Sum/1
  CGpos/1 -> Sum/2
  Sum/1 -> r x F/1
  Mux/1 -> r x F/2, Fprop/1
  Mux1/1 -> Sum2/1
  r x F/1 -> Sum2/2
  Sum2/1 -> Mprop/1

== system tp333079/FlightGear-Compatible/Propulsion/Tank ==
  Fuel Tank : Subsystem  SimViewingDevice=off  mask(Fuel Tank){MassIni=MassIni, Tank=Tank}
      mask prompts: MassIni "Initial mass:"; Tank "Tank structure:"
      mask help: The block integrates fuel flow to compute the tank inertia parameters.
      mask init:
      | if MassIni > Tank.Capacity
      | 	% Limit initial mass to tank capacity
      | 	MassIni = Tank.Capacity;
      | end
      settings: Permissions=ReadWrite  RTWFcnNameOpts=Auto  RTWFileNameOpts=Auto
      mask Help:
      | The block integrates fuel flow to compute the tank inertia parameters.
      | <P><B>Inputs:</B>
      | <LI>MassFlow = the current propellant mass flow (positive for propellant flowing out of the tank, negative otherwise)</LI>
      | <LI>RST = the flow integrator reset flag (integrator resets on rising edge)</LI>
      | </P>
      | <P><B>Outputs:</B>
      | <LI>Mass = the current mass of the propellant in the tank</LI>
      | <LI>CG = the tank CG location, in aircraft coordinates</LI>
      | <LI>Inertia = the tank moments of inertia [Jx Jy Jz Jxz]</LI>
      | </P>
      | <P><B>Parameters:</B>
      | <LI>Initial mass = the initial mass of propellant in the tank</LI>
      | <LI>Tank structure = the Matlab tank structure, part of the aircraft structure</LI>
      | </P>

== system tp333079/FlightGear-Compatible/Propulsion/Thruster ==
  Propeller : Subsystem  SimViewingDevice=off
      settings: Permissions=ReadWrite  RTWFcnNameOpts=Auto  RTWFileNameOpts=Auto

== system tp333079/Math/Normalization/Vector norm ==
  Vec : Inport  Port=1  PortDimensions=-1  SampleTime=-1  DataType=auto
      settings: SignalType=auto
  Dot Product : simulink3/Math/Dot Product
  Math Function : Math  Operator=sqrt  OutputSignalType=auto
  Mag : Outport  Port=1
  wires:
  Math Function/1 -> Mag/1
  Dot Product/1 -> Math Function/1
  Vec/1 -> Dot Product/2, Dot Product/1

== system tp333079/Math/Zero Offset/Non-zero Sign ==
  In : Inport  Port=1  PortDimensions=-1  SampleTime=-1  DataType=auto
      settings: SignalType=auto
  One : Constant  Value=1
  Relational Operator : RelationalOperator  Operator===
  Sign : Signum
  Switch : Switch  Threshold=1
  Zero : Constant  Value=0
  Out : Outport  Port=1
  wires:
  Zero/1 -> Relational Operator/2
  In/1 -> Relational Operator/1, Sign/1
  Relational Operator/1 -> Switch/2
  One/1 -> Switch/1
  Sign/1 -> Switch/3
  Switch/1 -> Out/1

== system tp333079/Propulsion/Piston Engine/Intake ==
  Thr : Inport  Port=1  PortDimensions=1  SampleTime=-1  DataType=double
      settings: SignalType=auto
  p : Inport  Port=2  PortDimensions=1  SampleTime=-1  DataType=double
      settings: SignalType=auto
  Get MAP : Product  Inputs=2  Multiplication=Element-wise(.*)  SaturateOnIntegerOverflow=on
  MAP min : Constant  Value=MAPmin
  Saturation : Saturate  UpperLimit=inf  LowerLimit=MAPmin  LinearizeAsGain=on
  Sum : Sum  Inputs=|+-  SaturateOnIntegerOverflow=on
  Sum1 : Sum  Inputs=|++  SaturateOnIntegerOverflow=on
  kPa : Gain  Gain=1/1000  Multiplication=Element-wise(K.*u)  SaturateOnIntegerOverflow=on
  MAP : Outport  Port=1
  wires:
  Saturation/1 -> MAP/1
  p/1 -> kPa/1
  Thr/1 -> Get MAP/1
  MAP min/1 -> Sum/2, Sum1/2
  kPa/1 -> Sum/1
  Sum/1 -> Get MAP/2
  Get MAP/1 -> Sum1/1
  Sum1/1 -> Saturation/1

== system tp333079/Sensors/Analog Sensors/A/D Converter ==
  Analog : Inport  Port=1  PortDimensions=-1  SampleTime=-1  DataType=auto
      settings: SignalType=auto
  Count size in Volts : Product  Inputs=*/  Multiplication=Element-wise(.*)  SaturateOnIntegerOverflow=on
  Max Counts : Constant  Value=2^Bits
  Max Volts : Constant  Value=MaxVolts
  Min Volts : Constant  Value=MinVolts
  Number of counts : Product  Inputs=*/  Multiplication=Element-wise(.*)  SaturateOnIntegerOverflow=on
  Rounding Function : Rounding  Operator=floor
  Saturation : Saturate  UpperLimit=2^Bits  LowerLimit=0  LinearizeAsGain=on
  Sum : Sum  Inputs=|+-  SaturateOnIntegerOverflow=on
  Sum1 : Sum  Inputs=|+-  SaturateOnIntegerOverflow=on
  Zero-Order Hold : ZeroOrderHold  SampleTime=tsamp
  Digital : Outport  Port=1
  wires:
  Zero-Order Hold/1 -> Digital/1
  Saturation/1 -> Zero-Order Hold/1
  Max Volts/1 -> Sum/1
  Min Volts/1 -> Sum/2, Sum1/2
  Max Counts/1 -> Count size in Volts/2
  Sum/1 -> Count size in Volts/1
  Analog/1 -> Sum1/1
  Sum1/1 -> Number of counts/1
  Count size in Volts/1 -> Number of counts/2
  Number of counts/1 -> Rounding Function/1
  Rounding Function/1 -> Saturation/1

== system tp333079/Sensors/Analog Sensors/Analog Sensor ==
  Input : Inport  Port=1  PortDimensions=1  SampleTime=-1  DataType=auto
      settings: SignalType=auto
  Bias Voltage : Constant  Value=BiasVolt
  Bias Point : Constant  Value=BiasPoint
  Scale Factor : Constant  Value=ScaleFactor
  Simple Sensor (2nd-order dynamics) : aerosimlib/Sensors/Generic Sensors/Simple Sensor (2nd-order dynamics)  MaxInput=Range(2)  MinInput=Range(1)  Bandwidth=Bandwidth  NoiseSeed=NoiseSeed  NoiseCov=NoiseCov  SampleTime=SampleTime
  Sum1 : Sum  Inputs=|++  SaturateOnIntegerOverflow=on
  Sum2 : Sum  Inputs=|+-  SaturateOnIntegerOverflow=on
  Unit conversion : Product  Inputs=2  Multiplication=Element-wise(.*)  SaturateOnIntegerOverflow=on
  Output : Outport  Port=1
  wires:
  Simple Sensor (2nd-order dynamics)/1 -> Sum2/1
  Bias Point/1 -> Sum2/2
  Sum2/1 -> Unit conversion/1
  Scale Factor/1 -> Unit conversion/2
  Unit conversion/1 -> Sum1/1
  Bias Voltage/1 -> Sum1/2
  Sum1/1 -> Output/1
  Input/1 -> Simple Sensor (2nd-order dynamics)/1

== system tp333079/Sensors/Digital Sensors/GPS PV ==
  PVIn : Inport  Port=1  PortDimensions=-1  SampleTime=-1  DataType=auto
      settings: SignalType=auto
  Altitude Measurement : aerosimlib/Sensors/Digital Sensors/Single GPS Measurement  ValIni=PosIni(3)  Lag=PosLag  TimeConst=TimeConst  seed=[32214]  Cov=VPosErr  T1=Trw
  Demux : Demux  Outputs=6  BusSelectionMode=off
  Latitude Measurement : aerosimlib/Sensors/Digital Sensors/Single GPS Measurement  ValIni=PosIni(1)  Lag=PosLag  TimeConst=TimeConst  seed=[44123]  Cov=HPosErr/REarth  T1=Trw
  Longitude Measurement : aerosimlib/Sensors/Digital Sensors/Single GPS Measurement  ValIni=PosIni(2)  Lag=PosLag  TimeConst=TimeConst  seed=[11243]  Cov=HPosErr/REarth  T1=Trw
  Mux : Mux  Inputs=6
  V Down Measurement : aerosimlib/Sensors/Digital Sensors/Single GPS Measurement  ValIni=VelIni(3)  Lag=VelLag  TimeConst=TimeConst  seed=[21143]  Cov=VVelErr  T1=Trw
  V East Measurement : aerosimlib/Sensors/Digital Sensors/Single GPS Measurement  ValIni=VelIni(2)  Lag=VelLag  TimeConst=TimeConst  seed=[43321]  Cov=HVelErr  T1=Trw
  V North Measurement : aerosimlib/Sensors/Digital Sensors/Single GPS Measurement  ValIni=VelIni(1)  Lag=VelLag  TimeConst=TimeConst  seed=[12344]  Cov=HVelErr  T1=Trw
  PVOut : Outport  Port=1
  wires:
  Demux/1 -> Latitude Measurement/1
  Demux/2 -> Longitude Measurement/1
  Demux/3 -> Altitude Measurement/1
  Demux/4 -> V North Measurement/1
  Demux/5 -> V East Measurement/1
  Demux/6 -> V Down Measurement/1
  PVIn/1 -> Demux/1
  Latitude Measurement/1 -> Mux/1
  Longitude Measurement/1 -> Mux/2
  Altitude Measurement/1 -> Mux/3
  V North Measurement/1 -> Mux/4
  V East Measurement/1 -> Mux/5
  V Down Measurement/1 -> Mux/6
  Mux/1 -> PVOut/1

== system tp333079/Sensors/Digital Sensors/Single GPS Measurement ==
  In : Inport  Port=1  PortDimensions=-1  SampleTime=-1  DataType=auto
      settings: SignalType=auto
  Gauss-Markov  Process : aerosimlib/Sensors/Noise Correlation/Gauss-Markov  Process  beta=TimeConst  seed=seed  Var=Cov^2  T=T1
  Sum : Sum  Inputs=|++  SaturateOnIntegerOverflow=on
  Transport Delay : TransportDelay  DelayTime=Lag  InitialInput=ValIni  BufferSize=1024  PadeOrder=0
  Out : Outport  Port=1
  wires:
  Sum/1 -> Out/1
  Gauss-Markov  Process/1 -> Sum/2
  In/1 -> Transport Delay/1
  Transport Delay/1 -> Sum/1

== system tp333079/Sensors/Generic Sensors/Simple Sensor (1st-order dynamics) ==
  Input : Inport  Port=1  PortDimensions=-1  SampleTime=-1  DataType=auto
      settings: SignalType=auto
  Random Walk : aerosimlib/Sensors/Noise Correlation/Random Walk  seed=NoiseSeed  Var=NoiseCov  T=SampleTime
  Saturation : Saturate  UpperLimit=MaxInput  LowerLimit=MinInput  LinearizeAsGain=on
  Sum : Sum  Inputs=|++  SaturateOnIntegerOverflow=on
  Transfer Fcn : TransferFcn  Numerator=[1]  Denominator=[Lag 1]  AbsoluteTolerance=auto  Realization=auto
  Output : Outport  Port=1
  wires:
  Sum/1 -> Output/1
  Random Walk/1 -> Sum/2
  Transfer Fcn/1 -> Sum/1
  Saturation/1 -> Transfer Fcn/1
  Input/1 -> Saturation/1

== system tp333079/Sensors/Generic Sensors/Simple Sensor (2nd-order dynamics) ==
  Input : Inport  Port=1  PortDimensions=-1  SampleTime=-1  DataType=auto
      settings: SignalType=auto
  Random Walk : aerosimlib/Sensors/Noise Correlation/Random Walk  seed=NoiseSeed  Var=NoiseCov  T=SampleTime
  Saturation : Saturate  UpperLimit=MaxInput  LowerLimit=MinInput  LinearizeAsGain=on
  Sum : Sum  Inputs=|++  SaturateOnIntegerOverflow=on
  Transfer Fcn : TransferFcn  Numerator=[wn^2]  Denominator=[1 2*zeta*wn wn^2]  AbsoluteTolerance=auto  Realization=auto
  Output : Outport  Port=1
  wires:
  Input/1 -> Saturation/1
  Saturation/1 -> Transfer Fcn/1
  Transfer Fcn/1 -> Sum/1
  Random Walk/1 -> Sum/2
  Sum/1 -> Output/1

== system tp333079/Sensors/Noise Correlation/Gauss-Markov  Process ==
  Gain : Gain  Orientation=left  Gain=1/beta  Multiplication=Element-wise(K.*u)  SaturateOnIntegerOverflow=on
  Integrator : Integrator  ExternalReset=none  InitialConditionSource=internal  InitialCondition=0  LimitOutput=off  UpperSaturationLimit=inf  LowerSaturationLimit=-inf  ShowSaturationPort=off  ShowStatePort=off  AbsoluteTolerance=auto
  Sum : Sum  Inputs=|+-  SaturateOnIntegerOverflow=on
  White Noise : RandomNumber  Mean=0  Variance=Var  Seed=seed  SampleTime=T
  Out : Outport  Port=1
  wires:
  Integrator/1 -> Out/1, Gain/1
  White Noise/1 -> Sum/1
  Sum/1 -> Integrator/1
  Gain/1 -> Sum/2

== system tp333079/Sensors/Noise Correlation/Random Walk ==
  Integrator : Integrator  ExternalReset=none  InitialConditionSource=internal  InitialCondition=0  LimitOutput=off  UpperSaturationLimit=inf  LowerSaturationLimit=-inf  ShowSaturationPort=off  ShowStatePort=off  AbsoluteTolerance=auto
  White Noise : RandomNumber  Mean=0  Variance=Var  Seed=seed  SampleTime=T
  Out : Outport  Port=1
  wires:
  White Noise/1 -> Integrator/1
  Integrator/1 -> Out/1

== system tp333079/Unit Conversion/Angular position/deg 2 rad ==
  In : Inport  Port=1  PortDimensions=-1  SampleTime=-1  DataType=auto
      settings: SignalType=auto
  Gain : Gain  Gain=pi/180  Multiplication=Element-wise(K.*u)  SaturateOnIntegerOverflow=on
  Out : Outport  Port=1
  wires:
  Gain/1 -> Out/1
  In/1 -> Gain/1

== system tp333079/Unit Conversion/Angular position/rad 2 deg ==
  In : Inport  Port=1  PortDimensions=-1  SampleTime=-1  DataType=auto
      settings: SignalType=auto
  Gain : Gain  Gain=180/pi  Multiplication=Element-wise(K.*u)  SaturateOnIntegerOverflow=on
  Out : Outport  Port=1
  wires:
  In/1 -> Gain/1
  Gain/1 -> Out/1

== system tp333079/Unit Conversion/Angular velocity/RPM 2 rad/s ==
  In : Inport  Port=1  PortDimensions=-1  SampleTime=-1  DataType=auto
      settings: SignalType=auto
  Gain : Gain  Gain=pi/30  Multiplication=Element-wise(K.*u)  SaturateOnIntegerOverflow=on
  Out : Outport  Port=1
  wires:
  In/1 -> Gain/1
  Gain/1 -> Out/1

== system tp333079/Unit Conversion/Angular velocity/rad/s 2 RPM ==
  In : Inport  Port=1  PortDimensions=-1  SampleTime=-1  DataType=auto
      settings: SignalType=auto
  Gain : Gain  Gain=30/pi  Multiplication=Element-wise(K.*u)  SaturateOnIntegerOverflow=on
  Out : Outport  Port=1
  wires:
  Gain/1 -> Out/1
  In/1 -> Gain/1

== system tp333079/Unit Conversion/Distance/ft 2 m ==
  In : Inport  Port=1  PortDimensions=-1  SampleTime=-1  DataType=auto
      settings: SignalType=auto
  Gain : Gain  Gain=0.3048  Multiplication=Element-wise(K.*u)  SaturateOnIntegerOverflow=on
  Out : Outport  Port=1
  wires:
  In/1 -> Gain/1
  Gain/1 -> Out/1

== system tp333079/Unit Conversion/Distance/m 2 ft ==
  In : Inport  Port=1  PortDimensions=-1  SampleTime=-1  DataType=auto
      settings: SignalType=auto
  Gain : Gain  Gain=1/0.3048  Multiplication=Element-wise(K.*u)  SaturateOnIntegerOverflow=on
  Out : Outport  Port=1
  wires:
  Gain/1 -> Out/1
  In/1 -> Gain/1

== system tp333079/Unit Conversion/Distance/m 2 nm ==
  In : Inport  Port=1  PortDimensions=-1  SampleTime=-1  DataType=auto
      settings: SignalType=auto
  Gain : Gain  Gain=1/1853.24496  Multiplication=Element-wise(K.*u)  SaturateOnIntegerOverflow=on
  Out : Outport  Port=1
  wires:
  In/1 -> Gain/1
  Gain/1 -> Out/1

== system tp333079/Unit Conversion/Distance/nm 2 m ==
  In : Inport  Port=1  PortDimensions=-1  SampleTime=-1  DataType=auto
      settings: SignalType=auto
  Gain : Gain  Gain=1853.24496  Multiplication=Element-wise(K.*u)  SaturateOnIntegerOverflow=on
  Out : Outport  Port=1
  wires:
  Gain/1 -> Out/1
  In/1 -> Gain/1

== system tp333079/Unit Conversion/Force/N 2 lbf ==
  In : Inport  Port=1  PortDimensions=-1  SampleTime=-1  DataType=auto
      settings: SignalType=auto
  Gain : Gain  Gain=0.22481  Multiplication=Element-wise(K.*u)  SaturateOnIntegerOverflow=on
  Out : Outport  Port=1
  wires:
  Gain/1 -> Out/1
  In/1 -> Gain/1

== system tp333079/Unit Conversion/Force/lbf 2 N ==
  In : Inport  Port=1  PortDimensions=-1  SampleTime=-1  DataType=auto
      settings: SignalType=auto
  Gain : Gain  Gain=1/0.22481  Multiplication=Element-wise(K.*u)  SaturateOnIntegerOverflow=on
  Out : Outport  Port=1
  wires:
  In/1 -> Gain/1
  Gain/1 -> Out/1

== system tp333079/Unit Conversion/Mass/kg 2 lb ==
  In : Inport  Port=1  PortDimensions=-1  SampleTime=-1  DataType=auto
      settings: SignalType=auto
  Gravity : Inport  Port=2  PortDimensions=-1  SampleTime=-1  DataType=auto
      settings: SignalType=auto
  Gain : Gain  Gain=0.22481  Multiplication=Element-wise(K.*u)  SaturateOnIntegerOverflow=on
  Product : Product  Inputs=2  Multiplication=Element-wise(.*)  SaturateOnIntegerOverflow=on
  Out : Outport  Port=1
  wires:
  Product/1 -> Gain/1
  Gravity/1 -> Product/2
  In/1 -> Product/1
  Gain/1 -> Out/1

== system tp333079/Unit Conversion/Mass/kg 2 slug ==
  In : Inport  Port=1  PortDimensions=-1  SampleTime=-1  DataType=auto
      settings: SignalType=auto
  Gain : Gain  Gain=0.068521  Multiplication=Element-wise(K.*u)  SaturateOnIntegerOverflow=on
  Out : Outport  Port=1
  wires:
  In/1 -> Gain/1
  Gain/1 -> Out/1

== system tp333079/Unit Conversion/Mass/lb 2 kg ==
  In : Inport  Port=1  PortDimensions=-1  SampleTime=-1  DataType=auto
      settings: SignalType=auto
  Gravity : Inport  Port=2  PortDimensions=-1  SampleTime=-1  DataType=auto
      settings: SignalType=auto
  Gain : Gain  Gain=1/0.22481  Multiplication=Element-wise(K.*u)  SaturateOnIntegerOverflow=on
  Product : Product  Inputs=*/  Multiplication=Element-wise(.*)  SaturateOnIntegerOverflow=on
  Out : Outport  Port=1
  wires:
  Product/1 -> Gain/1
  Gravity/1 -> Product/2
  In/1 -> Product/1
  Gain/1 -> Out/1

== system tp333079/Unit Conversion/Mass/slug 2 kg ==
  In : Inport  Port=1  PortDimensions=-1  SampleTime=-1  DataType=auto
      settings: SignalType=auto
  Gain : Gain  Gain=1/0.068521  Multiplication=Element-wise(K.*u)  SaturateOnIntegerOverflow=on
  Out : Outport  Port=1
  wires:
  Gain/1 -> Out/1
  In/1 -> Gain/1

== system tp333079/Unit Conversion/Pressure/Pa2inHg ==
  Pa : Inport  Port=1  PortDimensions=-1  SampleTime=-1  DataType=auto
      settings: SignalType=auto
  Gain : Gain  Gain=0.00029529  Multiplication=Element-wise(K.*u)  SaturateOnIntegerOverflow=on
  inHg : Outport  Port=1
  wires:
  Gain/1 -> inHg/1
  Pa/1 -> Gain/1
